simulink model "TV"  (R2023b)
settings: Solver=VariableStepAuto  StartTime=0.0  StopTime=6  RelTol=1e-3
libraries: simulink x2
settings Model: PacingRate=0.280000  Creator=joser  LastModifiedBy=joser

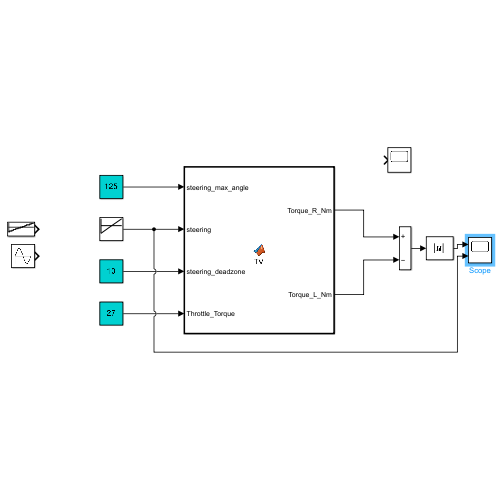
[thumbnail: Simulink's stored preview of the top-level diagram]
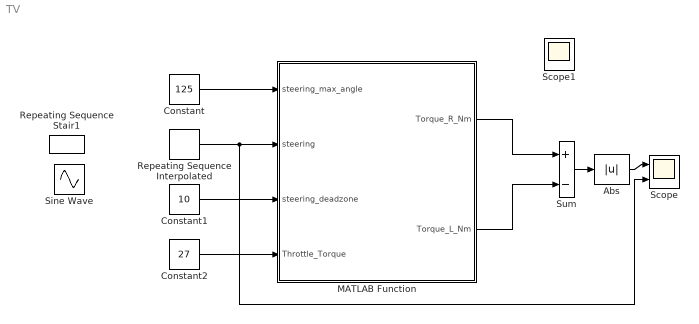
== system TV ==
  Abs : Abs  SaturateOnIntegerOverflow=off
  Constant : Constant  Value=125
  Constant1 : Constant  Value=10
  Constant2 : Constant  Value=27
  MATLAB Function : MATLAB Function  TreatAsAtomicUnit=on
  Repeating Sequence Interpolated : simulink/Sources/Repeating Sequence Interpolated  OutValues=[-125 0 125].'  TimeValues=[0 3 6].'  LookUpMeth=Interpolation-Use End Values  tsamp=0.01  OutMin=[]  OutMax=[]  OutDataTypeStr=double  OutputDataTypeScalingMode=double  OutDataType=fixdt(0,8)  OutScaling=2^-10
  Repeating Sequence Stair1 : simulink/Sources/Repeating Sequence Stair  OutValues=[-125, -120, -115, -110, -105, -100, -95, -90, -85, -80, -75, -70, -65, -60, -55, -50, -45, -40, -35, -30, -25, -20, -15, -10, -5, 0, 5, 10, 15, 20, 25, 30, 35, 40, 45, 50, 55, 60, 65, 70, 75, 80, 85, 90, 95, 100, 105, 110, 115, 120, 125]  tsamp=.025  OutMin=[]  OutMax=[]  OutDataTypeStr=double  OutputDataTypeScalingMode=double  OutDataType=fixdt(0,8)  ConRadixGroup=Best Precision: Vector-wise  OutScaling=2^-12
  Scope : Scope  NumInputPorts=2
  Scope1 : Scope
  Sine Wave : Sin  Amplitude=125  Frequency=pi/5  Phase=pi/2  SampleTime=0
  Sum : Sum  Inputs=+-
  wires:
  MATLAB Function/2(Torque_L_Nm) -> Sum/2
  Constant1/1 -> MATLAB Function/3(steering_deadzone)
  Constant2/1 -> MATLAB Function/4(Throttle_Torque)
  Constant/1 -> MATLAB Function/1(steering_max_angle)
  MATLAB Function/1(Torque_R_Nm) -> Sum/1
  Sum/1 -> Abs/1
  Abs/1 -> Scope/1
  Repeating Sequence Interpolated/1 -> Scope/2, MATLAB Function/2(steering)

== matlab function TV/MATLAB Function ==
  data: steering_max_angle input; Torque_R_Nm output; Torque_L_Nm output; steering input; steering_deadzone input; Throttle_Torque input
function [Torque_R_Nm, Torque_L_Nm] = TV(steering_max_angle, steering, steering_deadzone, Throttle_Torque)

if abs(steering) <= steering_deadzone % add steering deadzone (º)
    Torque_L_Nm = Throttle_Torque;
    Torque_R_Nm = Throttle_Torque;
    return;
end
d = (abs(steering) - steering_deadzone)/(steering_max_angle - steering_deadzone) * Throttle_Torque; %evaluate delta torque for given steering angle
if d > Throttle_Torque
     d = Throttle_Torque; %force torque to be positive to avoid balance issues
end
if steering < -steering_deadzone %if steering left, apply full torque to the emotor on the outside
       %and substract the delta from the inside one
    Torque_L_Nm = Throttle_Torque-d;
    Torque_R_Nm = Throttle_Torque;
    return;
else
%opposite case
Torque_L_Nm = Throttle_Torque;
Torque_R_Nm = Throttle_Torque-d;
return;
end
end
